simulink library "Pipe_stratified"  (Simulink 8.2)
settings: Solver=ode45  StartTime=0.0  StopTime=10.0  RelTol=1e-3
undefined symbols (not defined in the file): dia, height, nodes
libraries: carnot x1
settings Model: Creator=lena.frank  LastModifiedBy=drhf

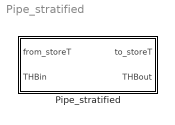
== system Pipe_stratified ==
  Pipe_stratified : Subsystem  mask(pipe connection to storage){h_in=0, h_out=0.8, nodes=nodes, hgt=height, dia=dia, dplin=0, dpqua=0}
      mask prompts: h_in "relative height of inlet"; h_out "relative height of outlet"; nodes "Number of nodes of storage (DO NOT CHANGE)"; hgt "Height vector (DO NOT CHANGE)"; dia "Diameter (DO NOT CHANGE)"; dplin "linear pressure drop"; dpqua "quadratic pressure drop"
      mask help:
      | The block transforms the incoming THV vector to a vector which the storage interprets as a flow into the storage fluid.
      | Give inlet- and outlet-height as a relative position from 0 (= bottom) to 1 (= top).
      mask init:
      | in = zeros(nodes,1);    % vector of length nodes
      | up = in;                % vector of length nodes
      | down = in;              % vector of length nodes
      | 
      | h_in = max(0,min(h_in,1));     % no nodes below 0 and above 1
      | h_out = max(0,min(h_out,1));   % no nodes below 0 and above 1
      | 
      | inlet = max(ceil(h_in*nodes),1);    % inlet position
      | outlet = max(ceil(h_out*nodes),1);  % outlet position
      | hgt = (h_out-h_in)*hgt;
      | 
      | in(inlet)=1;
      | 
      | 
      | idx_in_out = inlet:outlet;
      | if (inlet < outlet)             % if inlet below outlet
      |     up(inlet:outlet-1)=1;       % upwards
      |     n_concerned = inlet:outlet;
      |     flowdir = 1;
      | elseif (inlet > outlet)         % else if inlet above outlet
      |     down(outlet:inlet-1)=1;     % downwards
      |     n_concerned = outlet:inlet;
      |     idx_in_out = outlet:inlet;
      |     flowdir = -1;
      | end
      mask Help: web(fullfile(path_carnot('help'),'StoragePorts_PipeConnections.html'),'-helpbrowser')
      mask Display: disp('Pipe STRAT')

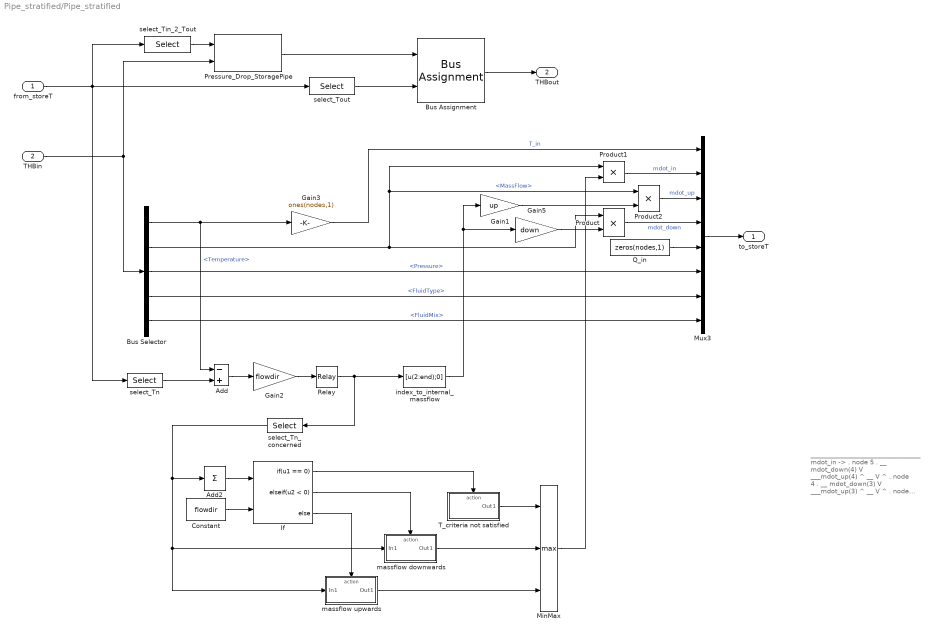
== system Pipe_stratified/Pipe_stratified ==
  note: _________________________________
      | mdot_in ->                                                .
      | node 5                     .
      | __ mdot_down(4) V  ___mdot_up(4) ^ __
      | V                           ^    .
      | node 4                    .
      | __ mdot_down(3) V  ___mdot_up(3) ^ __
      | V                           ^    .
      | node 3                    .
      | __ mdot_down(2) V  ___mdot_up(2) ^ __
      | V                           ^    .
      | node 2                    .
      | __ mdot_down(1) V  ___mdot_up(1) ^ __
      | V                           ^    .
      | node 1                    .
      | _________________________________
  from_storeT : Inport
  THBin : Inport  Port=2
  Add : Sum  Inputs=-+
  Add2 : Sum  Inputs=1
  Bus Assignment : BusAssignment  AssignedSignals=Temperature
  Bus Selector : BusSelector  OutputSignals=Temperature,MassFlow,Pressure,FluidType,FluidMix
  Constant : Constant  Value=flowdir
  Gain1 : Gain  Gain=up
  Gain2 : Gain  Gain=flowdir
  Gain3 : Gain  Gain=ones(nodes,1)
  Gain5 : Gain  Gain=down
  If : If  NumInputs=2  IfExpression=u1 == 0  ElseIfExpressions=u2 < 0
  MinMax : MinMax  Function=max  Inputs=3
  Mux3 : Mux  Inputs=8
  Pressure_Drop_StoragePipe : carnot/Basic/Pressure_Drop/Pressure_Drop_StoragePipe  dia=dia  hgt=hgt
  Product : Product  RndMeth=Zero
  Product1 : Product  RndMeth=Zero
  Product2 : Product  RndMeth=Zero
  Q_in : Constant  Value=zeros(nodes,1)
  Relay : Relay  OnSwitchValue=0.05  OffSwitchValue=-0.05
  T_criteria not satisfied : Subsystem  TreatAsAtomicUnit=on
  index_to_internal_massflow : MATLABFcn  MATLABFcn=[u(2:end);0]  OutputDimensions=nodes
  massflow downwards : Subsystem  TreatAsAtomicUnit=on
  massflow upwards : Subsystem  TreatAsAtomicUnit=on
  select_Tin_2_Tout : Selector  InputPortWidth=nodes  IndexOptions=Index vector (dialog)  Indices=[idx_in_out]  OutputSizes=1
  select_Tn : Selector  InputPortWidth=nodes  IndexOptions=Index vector (dialog)  Indices=[1:nodes]  OutputSizes=1
  select_Tn_concerned : Selector  InputPortWidth=nodes  IndexOptions=Index vector (dialog)  Indices=n_concerned  OutputSizes=1
  select_Tout : Selector  InputPortWidth=nodes  IndexOptions=Index vector (dialog)  Indices=[outlet]  OutputSizes=1
  to_storeT : Outport
  THBout : Outport  Port=2
  wires:
  index_to_internal_massflow/1 -> Gain1/1, Gain5/1
  Gain2/1 -> Relay/1
  massflow upwards/1(Out1) -> MinMax/3
  Product2/1 -> Mux3/3  "mdot_up"
  Gain1/1 -> Product2/2
  massflow downwards/1(Out1) -> MinMax/2
  If/3 -> massflow upwards/Action
  If/2 -> massflow downwards/Action
  T_criteria not satisfied/1(Out1) -> MinMax/1
  Constant/1 -> If/2
  If/1 -> T_criteria not satisfied/Action
  Add/1 -> Gain2/1
  select_Tn/1 -> Add/2
  Bus Selector/5 -> Mux3/8  "<FluidMix>"
  Bus Assignment/1 -> THBout/1
  Q_in/1 -> Mux3/5
  Gain3/1 -> Mux3/1  "T_in"
  select_Tout/1 -> Bus Assignment/2
  Mux3/1 -> to_storeT/1
  Bus Selector/1 -> Add/1, Gain3/1  "<Temperature>"
  Bus Selector/2 -> Product1/1, Product2/1, Product/1  "<MassFlow>"
  Bus Selector/3 -> Mux3/6  "<Pressure>"
  Bus Selector/4 -> Mux3/7  "<FluidType>"
  THBin/1 -> Bus Selector/1, Pressure_Drop_StoragePipe/2
  from_storeT/1 -> select_Tout/1, select_Tn/1, select_Tin_2_Tout/1
  Product/1 -> Mux3/4  "mdot_down"
  Relay/1 -> index_to_internal_massflow/1, select_Tn_concerned/1
  Gain5/1 -> Product/2
  Product1/1 -> Mux3/2  "mdot_in"
  Add2/1 -> If/1
  MinMax/1 -> Product1/2
  select_Tn_concerned/1 -> massflow upwards/1(In1), massflow downwards/1(In1), Add2/1
  Pressure_Drop_StoragePipe/1 -> Bus Assignment/1
  select_Tin_2_Tout/1 -> Pressure_Drop_StoragePipe/1

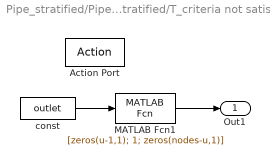
== system Pipe_stratified/Pipe_stratified/T_criteria not satisfied ==
  Action Port : ActionPort
  MATLAB Fcn1 : MATLABFcn  MATLABFcn=[zeros(u-1,1); 1; zeros(nodes-u,1)]  OutputDimensions=nodes
  const : Constant  Value=outlet
  Out1 : Outport  OutputWhenDisabled=reset  InitialOutput=0
  wires:
  MATLAB Fcn1/1 -> Out1/1
  const/1 -> MATLAB Fcn1/1

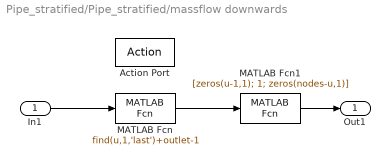
== system Pipe_stratified/Pipe_stratified/massflow downwards ==
  In1 : Inport
  Action Port : ActionPort
  MATLAB Fcn : MATLABFcn  MATLABFcn=find(u,1,'last')+outlet-1  OutputDimensions=1
  MATLAB Fcn1 : MATLABFcn  MATLABFcn=[zeros(u-1,1); 1; zeros(nodes-u,1)]  OutputDimensions=nodes
  Out1 : Outport
  wires:
  MATLAB Fcn1/1 -> Out1/1
  In1/1 -> MATLAB Fcn/1
  MATLAB Fcn/1 -> MATLAB Fcn1/1

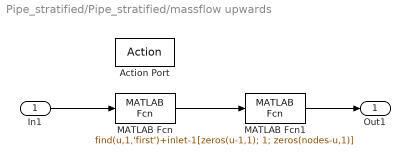
== system Pipe_stratified/Pipe_stratified/massflow upwards ==
  In1 : Inport
  Action Port : ActionPort
  MATLAB Fcn : MATLABFcn  MATLABFcn=find(u,1,'first')+inlet-1  OutputDimensions=1
  MATLAB Fcn1 : MATLABFcn  MATLABFcn=[zeros(u-1,1); 1; zeros(nodes-u,1)]  OutputDimensions=nodes
  Out1 : Outport
  wires:
  MATLAB Fcn1/1 -> Out1/1
  MATLAB Fcn/1 -> MATLAB Fcn1/1
  In1/1 -> MATLAB Fcn/1
